simulink model "Series_connected_PV_modules"  (Simulink 8.4)
settings: Solver=FixedStepDiscrete  StartTime=0.0  StopTime=1  FixedStep=1e-4  RelTol=1e-3
libraries: simulink x1
(part 2 of 2)

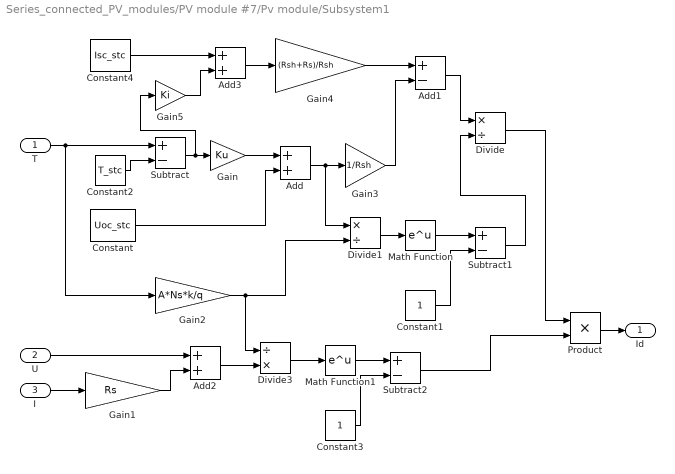
== system Series_connected_PV_modules/PV module #7/Pv module/Subsystem1 ==
  T : Inport
  U : Inport  Port=2
  I : Inport  Port=3
  Add : Sum
  Add1 : Sum  Inputs=+-
  Add2 : Sum
  Add3 : Sum
  Constant : Constant  Value=Uoc_stc
  Constant1 : Constant
  Constant2 : Constant  Value=T_stc
  Constant3 : Constant
  Constant4 : Constant  Value=Isc_stc
  Divide : Product  Inputs=*/
  Divide1 : Product  Inputs=*/
  Divide3 : Product  Inputs=/*
  Gain : Gain  Gain=Ku
  Gain1 : Gain  Gain=Rs
  Gain2 : Gain  Gain=A*Ns*k/q
  Gain3 : Gain  Gain=1/Rsh
  Gain4 : Gain  Gain=(Rsh+Rs)/Rsh
  Gain5 : Gain  Gain=Ki
  Math Function : Math  SaturateOnIntegerOverflow=on
  Math Function1 : Math  SaturateOnIntegerOverflow=on
  Product : Product  RndMeth=Zero
  Subtract : Sum  Inputs=+-
  Subtract1 : Sum  Inputs=+-
  Subtract2 : Sum  Inputs=+-
  Id : Outport
  wires:
  Constant4/1 -> Add3/1
  Constant2/1 -> Subtract/2
  T/1 -> Subtract/1, Gain2/1
  Add1/1 -> Divide/1
  Constant1/1 -> Subtract1/2
  Gain2/1 -> Divide1/2, Divide3/1
  Divide1/1 -> Math Function/1
  Math Function/1 -> Subtract1/1
  Subtract1/1 -> Divide/2
  Divide/1 -> Product/1
  U/1 -> Add2/1
  Add2/1 -> Divide3/2
  Divide3/1 -> Math Function1/1
  Math Function1/1 -> Subtract2/1
  Constant3/1 -> Subtract2/2
  Subtract2/1 -> Product/2
  Product/1 -> Id/1
  Add/1 -> Divide1/1, Gain3/1
  I/1 -> Gain1/1
  Gain1/1 -> Add2/2
  Gain3/1 -> Add1/2
  Gain5/1 -> Add3/2
  Add3/1 -> Gain4/1
  Gain/1 -> Add/1
  Constant/1 -> Add/2
  Subtract/1 -> Gain/1, Gain5/1
  Gain4/1 -> Add1/1

== system Series_connected_PV_modules/PV module #8/Bypass diode/Thermal voltage ==
  T : Inport
  Constant5 : Constant  Value=k/q
  Product : Product  RndMeth=Zero
  Vt : Outport
  wires:
  Product/1 -> Vt/1
  T/1 -> Product/1
  Constant5/1 -> Product/2

== system Series_connected_PV_modules/PV module #8/Pv module/Subsystem ==
  G : Inport
  T : Inport  Port=2
  Add : Sum
  Constant : Constant  Value=Isc_stc
  Constant1 : Constant  Value=T_stc
  Constant2 : Constant  Value=G_stc
  Divide : Product  Inputs=*/
  Gain : Gain  Gain=Ki
  Gain1 : Gain  Gain=(Rsh+Rs)/Rsh
  Product1 : Product  RndMeth=Zero
  Subtract : Sum  Inputs=+-
  Isc : Outport
  Ipv : Outport  Port=2
  wires:
  Gain1/1 -> Ipv/1
  Product1/1 -> Isc/1, Gain1/1
  Divide/1 -> Product1/2
  Add/1 -> Product1/1
  G/1 -> Divide/1
  T/1 -> Subtract/1
  Constant2/1 -> Divide/2
  Subtract/1 -> Gain/1
  Constant1/1 -> Subtract/2
  Gain/1 -> Add/2
  Constant/1 -> Add/1

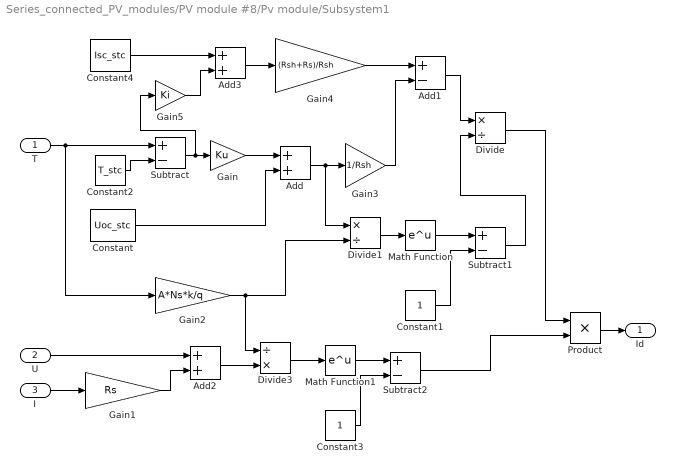
== system Series_connected_PV_modules/PV module #8/Pv module/Subsystem1 ==
  T : Inport
  U : Inport  Port=2
  I : Inport  Port=3
  Add : Sum
  Add1 : Sum  Inputs=+-
  Add2 : Sum
  Add3 : Sum
  Constant : Constant  Value=Uoc_stc
  Constant1 : Constant
  Constant2 : Constant  Value=T_stc
  Constant3 : Constant
  Constant4 : Constant  Value=Isc_stc
  Divide : Product  Inputs=*/
  Divide1 : Product  Inputs=*/
  Divide3 : Product  Inputs=/*
  Gain : Gain  Gain=Ku
  Gain1 : Gain  Gain=Rs
  Gain2 : Gain  Gain=A*Ns*k/q
  Gain3 : Gain  Gain=1/Rsh
  Gain4 : Gain  Gain=(Rsh+Rs)/Rsh
  Gain5 : Gain  Gain=Ki
  Math Function : Math  SaturateOnIntegerOverflow=on
  Math Function1 : Math  SaturateOnIntegerOverflow=on
  Product : Product  RndMeth=Zero
  Subtract : Sum  Inputs=+-
  Subtract1 : Sum  Inputs=+-
  Subtract2 : Sum  Inputs=+-
  Id : Outport
  wires:
  Gain4/1 -> Add1/1
  Subtract/1 -> Gain5/1, Gain/1
  Constant/1 -> Add/2
  Gain/1 -> Add/1
  Add3/1 -> Gain4/1
  Gain5/1 -> Add3/2
  Gain3/1 -> Add1/2
  Gain1/1 -> Add2/2
  I/1 -> Gain1/1
  Add/1 -> Gain3/1, Divide1/1
  Product/1 -> Id/1
  Subtract2/1 -> Product/2
  Constant3/1 -> Subtract2/2
  Math Function1/1 -> Subtract2/1
  Divide3/1 -> Math Function1/1
  Add2/1 -> Divide3/2
  U/1 -> Add2/1
  Divide/1 -> Product/1
  Subtract1/1 -> Divide/2
  Math Function/1 -> Subtract1/1
  Divide1/1 -> Math Function/1
  Gain2/1 -> Divide3/1, Divide1/2
  Constant1/1 -> Subtract1/2
  Add1/1 -> Divide/1
  T/1 -> Gain2/1, Subtract/1
  Constant2/1 -> Subtract/2
  Constant4/1 -> Add3/1

== system Series_connected_PV_modules/PV module #9/Bypass diode/Thermal voltage ==
  T : Inport
  Constant5 : Constant  Value=k/q
  Product : Product  RndMeth=Zero
  Vt : Outport
  wires:
  Constant5/1 -> Product/2
  T/1 -> Product/1
  Product/1 -> Vt/1

== system Series_connected_PV_modules/PV module #9/Pv module/Subsystem ==
  G : Inport
  T : Inport  Port=2
  Add : Sum
  Constant : Constant  Value=Isc_stc
  Constant1 : Constant  Value=T_stc
  Constant2 : Constant  Value=G_stc
  Divide : Product  Inputs=*/
  Gain : Gain  Gain=Ki
  Gain1 : Gain  Gain=(Rsh+Rs)/Rsh
  Product1 : Product  RndMeth=Zero
  Subtract : Sum  Inputs=+-
  Isc : Outport
  Ipv : Outport  Port=2
  wires:
  Constant/1 -> Add/1
  Gain/1 -> Add/2
  Constant1/1 -> Subtract/2
  Subtract/1 -> Gain/1
  Constant2/1 -> Divide/2
  T/1 -> Subtract/1
  G/1 -> Divide/1
  Add/1 -> Product1/1
  Divide/1 -> Product1/2
  Product1/1 -> Gain1/1, Isc/1
  Gain1/1 -> Ipv/1

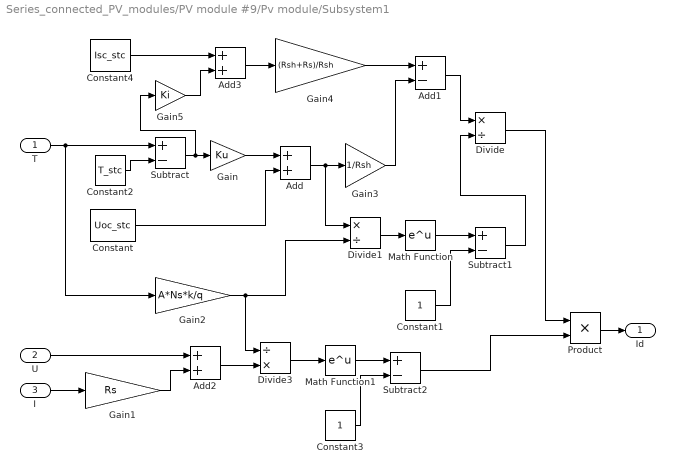
== system Series_connected_PV_modules/PV module #9/Pv module/Subsystem1 ==
  T : Inport
  U : Inport  Port=2
  I : Inport  Port=3
  Add : Sum
  Add1 : Sum  Inputs=+-
  Add2 : Sum
  Add3 : Sum
  Constant : Constant  Value=Uoc_stc
  Constant1 : Constant
  Constant2 : Constant  Value=T_stc
  Constant3 : Constant
  Constant4 : Constant  Value=Isc_stc
  Divide : Product  Inputs=*/
  Divide1 : Product  Inputs=*/
  Divide3 : Product  Inputs=/*
  Gain : Gain  Gain=Ku
  Gain1 : Gain  Gain=Rs
  Gain2 : Gain  Gain=A*Ns*k/q
  Gain3 : Gain  Gain=1/Rsh
  Gain4 : Gain  Gain=(Rsh+Rs)/Rsh
  Gain5 : Gain  Gain=Ki
  Math Function : Math  SaturateOnIntegerOverflow=on
  Math Function1 : Math  SaturateOnIntegerOverflow=on
  Product : Product  RndMeth=Zero
  Subtract : Sum  Inputs=+-
  Subtract1 : Sum  Inputs=+-
  Subtract2 : Sum  Inputs=+-
  Id : Outport
  wires:
  Constant4/1 -> Add3/1
  Constant2/1 -> Subtract/2
  T/1 -> Subtract/1, Gain2/1
  Add1/1 -> Divide/1
  Constant1/1 -> Subtract1/2
  Gain2/1 -> Divide1/2, Divide3/1
  Divide1/1 -> Math Function/1
  Math Function/1 -> Subtract1/1
  Subtract1/1 -> Divide/2
  Divide/1 -> Product/1
  U/1 -> Add2/1
  Add2/1 -> Divide3/2
  Divide3/1 -> Math Function1/1
  Math Function1/1 -> Subtract2/1
  Constant3/1 -> Subtract2/2
  Subtract2/1 -> Product/2
  Product/1 -> Id/1
  Add/1 -> Divide1/1, Gain3/1
  I/1 -> Gain1/1
  Gain1/1 -> Add2/2
  Gain3/1 -> Add1/2
  Gain5/1 -> Add3/2
  Add3/1 -> Gain4/1
  Gain/1 -> Add/1
  Constant/1 -> Add/2
  Subtract/1 -> Gain/1, Gain5/1
  Gain4/1 -> Add1/1
